simulink model "nonlinear_ss_control_reg"  (R2019b)
settings: Solver=ode45  StartTime=0.0  StopTime=1500.0  MaxStep=0.001  RelTol=1e-8
settings Model: Creator=Hector  LastModifiedBy=Hector

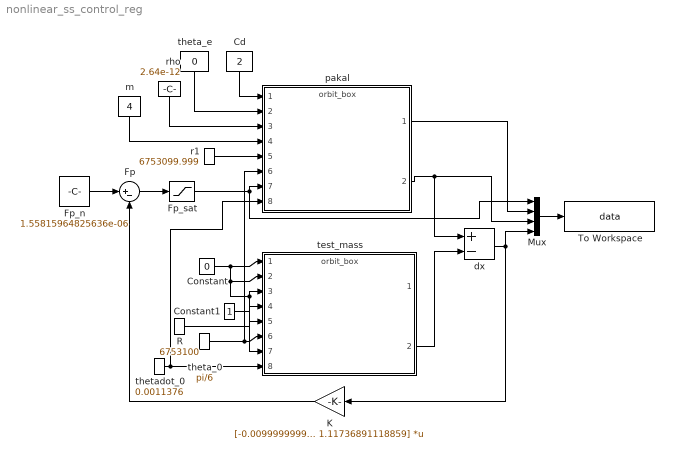
== system nonlinear_ss_control_reg ==
  Cd : Constant  Value=2
  Constant : Constant  Value=0
  Constant1 : Constant
  Fp : Sum  Inputs=|+-
  Fp_n : Constant  Value=1.55815964825636e-06
  Fp_sat : Saturate  UpperLimit=2e-05  LowerLimit=0
  K : Gain  Gain=[-0.00999999999175389 963078.643670276 0.0102433611048443 1.11736891118859]  Multiplication=Matrix(K*u)
  Mux : Mux
  R : Constant  Value=6753100
  To Workspace : ToWorkspace  VariableName=data  SaveFormat=Timeseries  SampleTime=-1
  dx : Sum  Inputs=+-
  m : Constant  Value=4
  pakal : ModelReference  ModelNameDialog=orbit_box.slx  SimulationMode=Normal  ModelReferenceVersion=1.40
  r1 : Constant  Value=6753099.999
  rho : Constant  Value=2.64e-12
  test_mass : ModelReference  ModelNameDialog=orbit_box.slx  SimulationMode=Normal  ModelReferenceVersion=1.40
  theta_0 : Constant  Value=pi/6
  theta_e : Constant  Value=0
  thetadot_0 : Constant  Value=0.0011376
  wires:
  Fp_n/1 -> Fp/1
  R/1 -> test_mass/5
  Constant1/1 -> test_mass/4
  r1/1 -> pakal/5
  m/1 -> pakal/4
  rho/1 -> pakal/3
  theta_e/1 -> pakal/2
  Cd/1 -> pakal/1
  Mux/1 -> To Workspace/1
  Fp/1 -> Fp_sat/1
  Fp_sat/1 -> Mux/1, pakal/7
  K/1 -> Fp/2
  theta_0/1 -> pakal/6, test_mass/6
  Constant/1 -> test_mass/7, test_mass/3, test_mass/2, test_mass/1
  test_mass/2 -> dx/2
  dx/1 -> K/1, Mux/4
  pakal/1 -> Mux/2
  pakal/2 -> dx/1, Mux/3
  thetadot_0/1 -> pakal/8, test_mass/8
